simulink model "NNModel"  (R2019a)
settings: Solver=ode4  StartTime=0.0  StopTime=3  FixedStep=.01  MaxStep=.001  RelTol=1e-3  EnableMultiTasking=on
settings Model: Creator=X_501  LastModifiedBy=HUAWEI-PC
settings DataIOCC: LimitDataPoints=on  SaveFormat=Array  ReturnWorkspaceOutputs=off
settings OptimizationCC: LifeSpan=inf
settings DebuggingCC: SFUnexpectedBacktrackingDiag=warning  SFNoUnconditionalDefaultTransitionDiag=warning  SFExecutionAtInitializationDiag=none  ArithmeticOperatorsInVariantConditions=warning
settings HardwareCC: ProdBitPerPointer=32  ProdBitPerSizeT=32  ProdBitPerPtrDiffT=32  ProdLargestAtomicFloat=None  ProdIntDivRoundTo=Undefined  ProdEndianess=Unspecified  ProdWordSize=32  ProdHWDeviceType=32-bit Generic
settings ModelReferenceCC: PropagateSignalLabelsOutOfModel=off
settings SFSimCC: SimUseLocalCustomCode=off
settings RTWCC: RTWUseLocalCustomCode=off
settings CodeAppCC: StateflowObjectComments=on
settings GRTTargetCC: TargetLangStandard=C89/C90 (ANSI)  GeneratePreprocessorConditionals=Disable all
settings ConfigComp: CovMetricSettings=dw  CovHtmlReporting=on  CovSaveCumulativeToWorkspaceVar=on  CovSaveSingleToWorkspaceVar=on  CovExternalEMLEnable=off

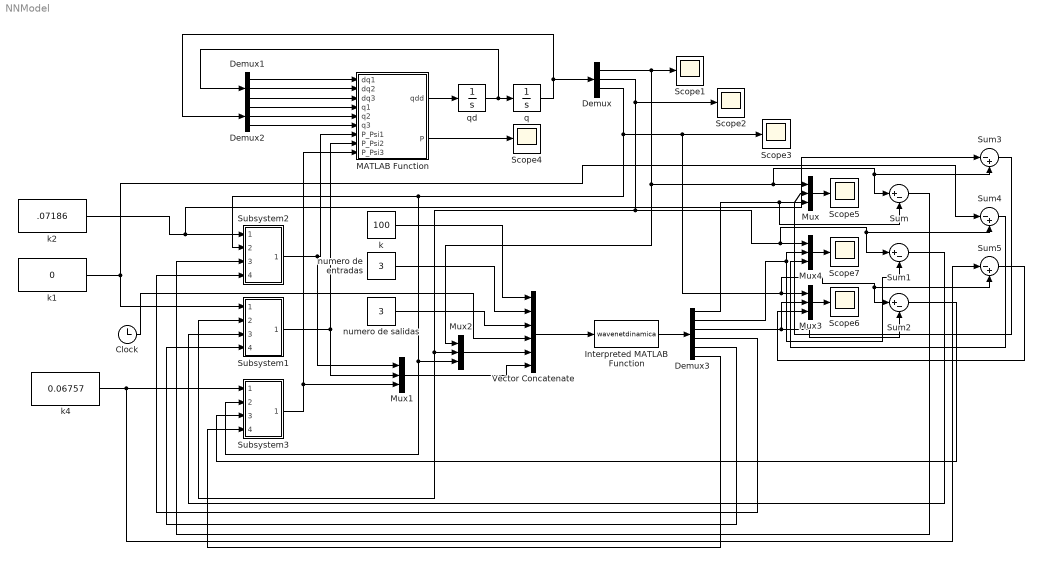
== system NNModel ==
  Clock : Clock
      settings: Decimation=40
  Demux : Demux  Outputs=3
  Demux1 : Demux  Outputs=3
  Demux2 : Demux  Outputs=3
  Demux3 : Demux  Outputs=6
  Interpreted MATLAB Function : MATLABFcn  MATLABFcn=wavenetdinamica  OutputDimensions=6
  MATLAB Function : MATLAB Function  TreatAsAtomicUnit=on
  Mux{,1..4} (5 alike) : Mux  Inputs=3
  Scope{1..7} (7 alike) : Scope
  Subsystem1 : Subsystem
  Subsystem2 : Subsystem
  Subsystem3 : Subsystem
  Sum : Sum  Inputs=|+-
  Sum1 : Sum  Inputs=|+-
  Sum2 : Sum  Inputs=|+-
  Sum3 : Sum  Inputs=|-+
  Sum4 : Sum  Inputs=|-+
  Sum5 : Sum  Inputs=|-+
  Vector Concatenate : Concatenate  NumInputs=6
  k : Constant  Value=100
  k1 : Constant  Value=0
  k2 : Constant  Value=.07186
  k4 : Constant  Value=0.06757
  numero de entradas : Constant  Value=3
  numero de salidas : Constant  Value=3
  q : Integrator  InitialCondition=[0.0718;0;0.0675]
  qd : Integrator  InitialCondition=[0;0;0]
  wires:
  MATLAB Function/1(qdd) -> qd/1
  qd/1 -> q/1, Demux1/1
  q/1 -> Demux2/1, Demux/1
  Demux/1 -> Mux2/1, Sum3/2, Sum/1, Mux/1, Scope1/1
  Demux1/1 -> MATLAB Function/1(dq1)
  Demux1/2 -> MATLAB Function/2(dq2)
  Demux1/3 -> MATLAB Function/3(dq3)
  Demux2/1 -> MATLAB Function/4(q1)
  Demux2/2 -> MATLAB Function/5(q2)
  Demux2/3 -> MATLAB Function/6(q3)
  MATLAB Function/2(P) -> Scope4/1
  Vector Concatenate/1 -> Interpreted MATLAB Function/1
  Mux/1 -> Scope5/1
  k/1 -> Vector Concatenate/1
  numero de entradas/1 -> Vector Concatenate/2
  Clock/1 -> Vector Concatenate/4
  numero de salidas/1 -> Vector Concatenate/3
  Mux3/1 -> Scope6/1
  Interpreted MATLAB Function/1 -> Demux3/1
  Demux/3 -> Mux2/3, Subsystem3/2(In2), Subsystem2/2(In2), Sum5/2, Sum2/1, Mux3/1, Scope3/1
  Demux3/1 -> Sum/2, Mux/2
  Demux/2 -> Scope2/1, Subsystem1/2(In2), Mux2/2, Sum4/2, Sum1/1, Mux4/1
  Demux3/3 -> Sum2/2, Mux3/2
  Mux4/1 -> Scope7/1
  Demux3/2 -> Sum1/2, Mux4/2
  k2/1 -> Sum3/1, Subsystem2/1(In1)
  Subsystem2/1(Out1) -> Mux1/1, MATLAB Function/7(P_Psi1)
  Subsystem1/1(Out1) -> MATLAB Function/8(P_Psi2), Mux1/2
  Demux3/4 -> Subsystem2/4(In4)
  Demux3/5 -> Subsystem1/4(In4)
  Sum/1 -> Subsystem2/3(In3)
  Sum1/1 -> Subsystem1/3(In3)
  k1/1 -> Subsystem1/1(In1), Sum4/1
  Subsystem3/1(Out1) -> Mux1/3, MATLAB Function/9(P_Psi3)
  Demux3/6 -> Subsystem3/4(In4)
  Sum2/1 -> Subsystem3/3(In3)
  k4/1 -> Sum5/1, Subsystem3/1(In1)
  Mux2/1 -> Vector Concatenate/5
  Mux1/1 -> Vector Concatenate/6
  Sum3/1 -> Mux/3
  Sum4/1 -> Mux4/3
  Sum5/1 -> Mux3/3

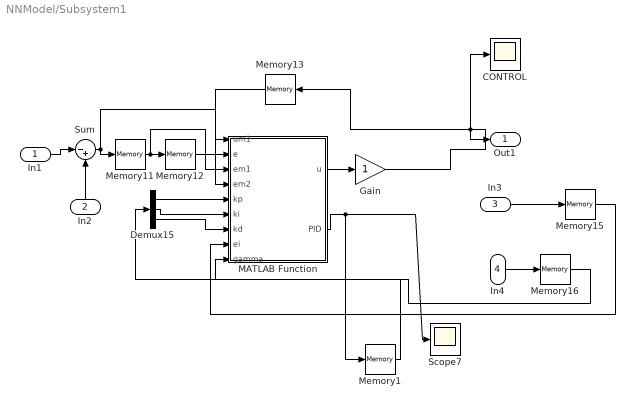
== system NNModel/Subsystem1 ==
  In1 : Inport
  In2 : Inport  Port=2
  In3 : Inport  Port=3
  In4 : Inport  Port=4
  CONTROL : Scope
  Demux15 : Demux  Outputs=3
  Gain : Gain
  MATLAB Function : MATLAB Function  TreatAsAtomicUnit=on
  Memory1 : Memory  InitialCondition=[.1;1;0]
  Memory{11..13,15..16} (5 alike) : Memory
  Scope7 : Scope
  Sum : Sum  Inputs=|-+
  Out1 : Outport
  wires:
  Memory16/1 -> MATLAB Function/9(gamma)
  Memory15/1 -> MATLAB Function/8(ei)
  Gain/1 -> Memory13/1, CONTROL/1, Out1/1
  Demux15/3 -> MATLAB Function/7(kd)
  Demux15/2 -> MATLAB Function/6(ki)
  Demux15/1 -> MATLAB Function/5(kp)
  Memory1/1 -> Demux15/1
  MATLAB Function/2(PID) -> Scope7/1, Memory1/1
  Memory12/1 -> MATLAB Function/4(em2)
  Memory13/1 -> MATLAB Function/1(um1)
  MATLAB Function/1(u) -> Gain/1
  Memory11/1 -> Memory12/1, MATLAB Function/3(em1)
  Sum/1 -> Memory11/1, MATLAB Function/2(e)
  In2/1 -> Sum/2
  In3/1 -> Memory15/1
  In4/1 -> Memory16/1
  In1/1 -> Sum/1

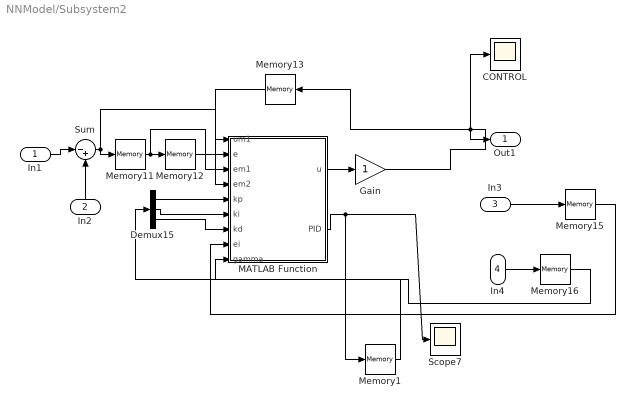
== system NNModel/Subsystem2 ==
  In1 : Inport
  In2 : Inport  Port=2
  In3 : Inport  Port=3
  In4 : Inport  Port=4
  CONTROL : Scope
  Demux15 : Demux  Outputs=3
  Gain : Gain
  MATLAB Function : MATLAB Function  TreatAsAtomicUnit=on
  Memory1 : Memory  InitialCondition=[.1;0;0]
  Memory{11..13,15..16} (5 alike) : Memory
  Scope7 : Scope
  Sum : Sum  Inputs=|-+
  Out1 : Outport
  wires:
  In1/1 -> Sum/1
  In4/1 -> Memory16/1
  In3/1 -> Memory15/1
  In2/1 -> Sum/2
  Sum/1 -> MATLAB Function/2(e), Memory11/1
  Memory11/1 -> MATLAB Function/3(em1), Memory12/1
  MATLAB Function/1(u) -> Gain/1
  Memory13/1 -> MATLAB Function/1(um1)
  Memory12/1 -> MATLAB Function/4(em2)
  MATLAB Function/2(PID) -> Memory1/1, Scope7/1
  Memory1/1 -> Demux15/1
  Demux15/1 -> MATLAB Function/5(kp)
  Demux15/2 -> MATLAB Function/6(ki)
  Demux15/3 -> MATLAB Function/7(kd)
  Gain/1 -> Out1/1, CONTROL/1, Memory13/1
  Memory15/1 -> MATLAB Function/8(ei)
  Memory16/1 -> MATLAB Function/9(gamma)

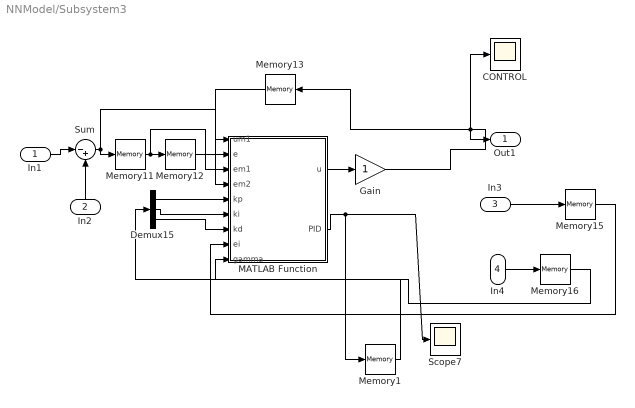
== system NNModel/Subsystem3 ==
  In1 : Inport
  In2 : Inport  Port=2
  In3 : Inport  Port=3
  In4 : Inport  Port=4
  CONTROL : Scope
  Demux15 : Demux  Outputs=3
  Gain : Gain
  MATLAB Function : MATLAB Function  TreatAsAtomicUnit=on
  Memory1 : Memory  InitialCondition=[1;0;0]
  Memory{11..13,15..16} (5 alike) : Memory
  Scope7 : Scope
  Sum : Sum  Inputs=|-+
  Out1 : Outport
  wires:
  In1/1 -> Sum/1
  In4/1 -> Memory16/1
  In3/1 -> Memory15/1
  In2/1 -> Sum/2
  Sum/1 -> MATLAB Function/2(e), Memory11/1
  Memory11/1 -> MATLAB Function/3(em1), Memory12/1
  MATLAB Function/1(u) -> Gain/1
  Memory13/1 -> MATLAB Function/1(um1)
  Memory12/1 -> MATLAB Function/4(em2)
  MATLAB Function/2(PID) -> Memory1/1, Scope7/1
  Memory1/1 -> Demux15/1
  Demux15/1 -> MATLAB Function/5(kp)
  Demux15/2 -> MATLAB Function/6(ki)
  Demux15/3 -> MATLAB Function/7(kd)
  Gain/1 -> Out1/1, CONTROL/1, Memory13/1
  Memory15/1 -> MATLAB Function/8(ei)
  Memory16/1 -> MATLAB Function/9(gamma)

== matlab function NNModel/Subsystem1/MATLAB Function ==
  data: um1 input; e input; u output; em1 input; em2 input; kp input; ki input; kd input; PID output; ei input; gamma input
function [u, PID] = fcn(um1, e, em1, em2, kp, ki, kd, ei, gamma)
T=0.01;
Ti=kp/ki;
Td=kd/kp;

k0=kp*(1+(T/Ti)+(Td/T));
k1=-kp*(1+2*(Td/T));
k2=kp*(Td/T);


u = um1+ k0*e + k1*em1 + k2*em2;

miup=.05;
miui=.05;
miud=1000.555;

% nkp=kp;
% nki=ki;
% nkd=kd;
nkp=kp+miup*ei*gamma*(e-em1)
nki=ki+miui*ei*gamma*e
nkd=kd+miud*ei*gamma*(e-2*em1+em2)

PID=[nkp; nki; nkd];

== matlab function NNModel/MATLAB Function ==
  data: dq1 input; dq2 input; dq3 input; qdd output; q1 input; q2 input; q3 input; P_Psi1 input; P output; P_Psi2 input; P_Psi3 input
function [qdd,P]  = fcn(dq1,dq2,dq3,q1,q2,q3,P_Psi1,P_Psi2,P_Psi3)
% Parametros 
q = [q1 q2 q3]';
dq = [dq1 dq2 dq3]';

% Parametros constantes
l0=0.085;     % Longitud inicial
rm = 0.008;  % Radio hacia las camaras
rch = 0.00175;  % Radio de las camaras
qi = [l0 0 0.05]';

% Variables de deformación
l=q(1); phi=q(2); k=q(3);

% Presión de Entrada
fc = 6894.76; % Factor de conversión de Psi a Pascal
% Presion de entrada transformada a unidades de pascal
P = [P_Psi1*fc;P_Psi2*fc;P_Psi3*fc]; 

% Matriz de Inercia
H = M_Inercia_d(q);
% Matriz de Coriolis
C = Coriolis_d(q,dq);
% Vector de gravedad
gq = gr_d(q);

% Matriz de elasticidad lineal
Ke = [20.3077 0       0;
        0     0       0;
        0      0  6.3459e-05];
% Matriz de disipacion
D = diag([2e-2 0 2e-6]); 
% Fuerza elastica
Fe = Ke*(q-qi); 
% Fuerzas disipativas
Fd = D*dq; 

% Matriz de entrada
Bv = [ -pi*rch^2*(k*rm*cos(phi) - 1),            pi*k*l*rm*rch^2*sin(phi),       -pi*l*rm*rch^2*cos(phi);
     rch^2*pi*(k*rm*cos(phi + pi/3) + 1),    -k*l*rm*rch^2*pi*sin(phi + pi/3), l*rm*rch^2*pi*cos(phi + pi/3);
     rch^2*pi*(k*rm*sin(phi + pi/6) + 1), k*l*rm*rch^2*pi*sin(phi + (2*pi)/3), l*rm*rch^2*pi*sin(phi + pi/6)]';
% Pares generalizados generados por presion
taup = Bv*P;
% Resolver para aceleracion
qdd = inv(H)*(taup-C*dq-gq-Fe-Fd);
end

== matlab function NNModel/Subsystem3/MATLAB Function ==
  data: um1 input; e input; u output; em1 input; em2 input; kp input; ki input; kd input; PID output; ei input; gamma input
function [u, PID] = fcn(um1, e, em1, em2, kp, ki, kd, ei, gamma)
T=0.01;
Ti=kp/ki;
Td=kd/kp;

k0=kp*(1+(T/Ti)+(Td/T));
k1=-kp*(1+2*(Td/T));
k2=kp*(Td/T);


u = um1+ k0*e + k1*em1 + k2*em2;

miup=.05;
miui=.05;
miud=.5;

% nkp=kp;
% nki=ki;
% nkd=kd;
nkp=kp+miup*ei*gamma*(e-em1)
nki=ki+miui*ei*gamma*e
nkd=kd+miud*ei*gamma*(e-2*em1+em2)

PID=[nkp; nki; nkd];

== matlab function NNModel/Subsystem2/MATLAB Function ==
  data: um1 input; e input; u output; em1 input; em2 input; kp input; ki input; kd input; PID output; ei input; gamma input
function [u, PID] = fcn(um1, e, em1, em2, kp, ki, kd, ei, gamma)
T=0.01;
Ti=kp/ki;
Td=kd/kp;

k0=kp*(1+(T/Ti)+(Td/T));
k1=-kp*(1+2*(Td/T));
k2=kp*(Td/T);


u = um1+ k0*e + k1*em1 + k2*em2;

miup=.05;
miui=.05;
miud=.5;

% nkp=kp;
% nki=ki;
% nkd=kd;
nkp=kp+miup*ei*gamma*(e-em1)
nki=ki+miui*ei*gamma*e
nkd=kd+miud*ei*gamma*(e-2*em1+em2)

PID=[nkp; nki; nkd];
